simulink model "test_SOC_single_cell"  (R2024a)
settings: Solver=FixedStepAuto  StartTime=0.0  StopTime=.2  FixedStep=.01  RelTol=1e-3
values from neighbouring files (symbols this model uses):
  SOX_Ts = 1.0    [ParametersDataDictionary.sldd]
libraries: simulink x4
settings Model: DataDictionary=ParametersDataDictionaryGotion.sldd  Creator=mmackenzie  LastModifiedBy=mmackenzie
settings DebuggingCC: ParamPrecisionLossAbsoluteDiffThreshold=1e-10  ParamPrecisionLossRelativeDiffThreshold=1e-7

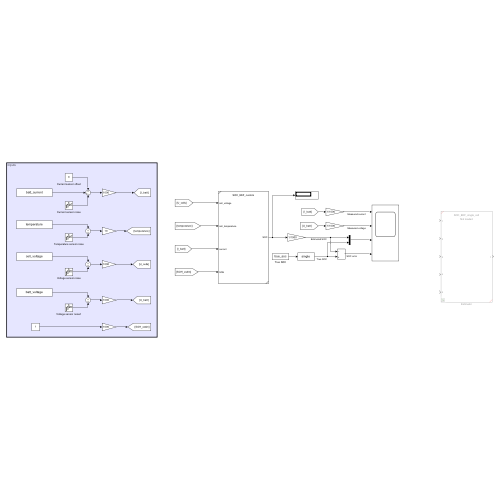
[thumbnail: Simulink's stored preview of the top-level diagram]
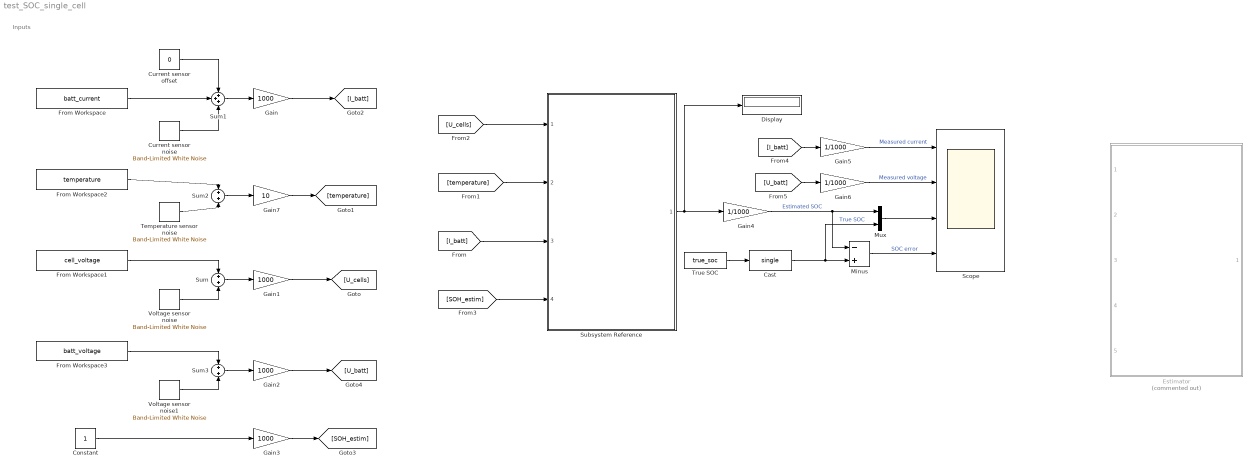
== system test_SOC_single_cell ==
  note: Inputs
  Cast : DataTypeConversion  OutDataTypeStr=single  SaturateOnIntegerOverflow=off  RndMeth=Floor
  Constant : Constant
  Current sensor noise : simulink/Sources/Band-Limited White Noise  Cov=.001  Ts=1  seed=42
  Current sensor offset : Constant  Value=0
  Display : Display
  Estimator : Subsystem  Commented=on  ReferencedSubsystem=SOC_EKF_single_cell
      settings: PermitHierarchicalResolution=None
  From Workspace : FromWorkspace  VariableName=batt_current
  From Workspace1 : FromWorkspace  VariableName=cell_voltage
  From Workspace2 : FromWorkspace  VariableName=temperature
  From Workspace3 : FromWorkspace  VariableName=batt_voltage
  Gain{,1..3} (4 alike) : Gain  Gain=1000
  Gain4 : Gain  Gain=1/1000
  Gain5 : Gain  Gain=1/1000
  Gain6 : Gain  Gain=1/1000
  Gain7 : Gain  Gain=10
  Minus : Sum  Inputs=-+
  Mux : Mux  Inputs=2
  Scope : Scope  NumInputPorts=4
  Subsystem Reference : Subsystem  ReferencedSubsystem=SOC_EKF_custom
      settings: PermitHierarchicalResolution=None
  Sum : Sum
  Sum1 : Sum  Inputs=+++
  Sum2 : Sum
  Sum3 : Sum
  Temperature sensor noise : simulink/Sources/Band-Limited White Noise  Cov=1  Ts=SOX_Ts  seed=42
  True SOC : FromWorkspace  VariableName=true_soc
  Voltage sensor noise : simulink/Sources/Band-Limited White Noise  Cov=1e-6  Ts=SOX_Ts  seed=42
  Voltage sensor noise1 : simulink/Sources/Band-Limited White Noise  Cov=1e-6  Ts=SOX_Ts  seed=42
  wires:
  Subsystem Reference/1 -> Display/1, Gain4/1
  From Workspace1/1 -> Sum/1
  Voltage sensor noise/1 -> Sum/2
  Sum/1 -> Gain1/1
  From Workspace2/1 -> Sum2/1
  Temperature sensor noise/1 -> Sum2/2
  Sum2/1 -> Gain7/1
  From Workspace/1 -> Sum1/2
  Current sensor noise/1 -> Sum1/3
  Current sensor offset/1 -> Sum1/1
  Sum1/1 -> Gain/1
  Constant/1 -> Gain3/1
  [I_batt] -> Gain5/1
  [U_batt] -> Gain6/1
  Mux/1 -> Scope/3
  Minus/1 -> Scope/4  "SOC error"
  [temperature] -> Subsystem Reference/2
  [I_batt] -> Subsystem Reference/3
  [SOH_estim] -> Subsystem Reference/4
  Sum3/1 -> Gain2/1
  Voltage sensor noise1/1 -> Sum3/2
  From Workspace3/1 -> Sum3/1
  [U_cells] -> Subsystem Reference/1
  True SOC/1 -> Cast/1
  Cast/1 -> Minus/2, Mux/2  "True SOC"
  Gain/1 -> [I_batt]
  Gain1/1 -> [U_cells]
  Gain2/1 -> [U_batt]
  Gain3/1 -> [SOH_estim]
  Gain7/1 -> [temperature]
  Gain4/1 -> Minus/1, Mux/1  "Estimated SOC"
  Gain5/1 -> Scope/1  "Measured current"
  Gain6/1 -> Scope/2  "Measured voltage"
